simulink model "main_commande"  (R2024b)
settings: Solver=FixedStepAuto  StartTime=0.0  StopTime=10.0  MaxStep=0.01  RelTol=1e-3
undefined symbols (not defined in the file or in its folder): Cf, Cr, e_max, epsilon, Izz, lf, lr, m, q, TV
libraries: simulink x2
settings Model: PacingRate=0.100000  Creator=marti  LastModifiedBy=Filip

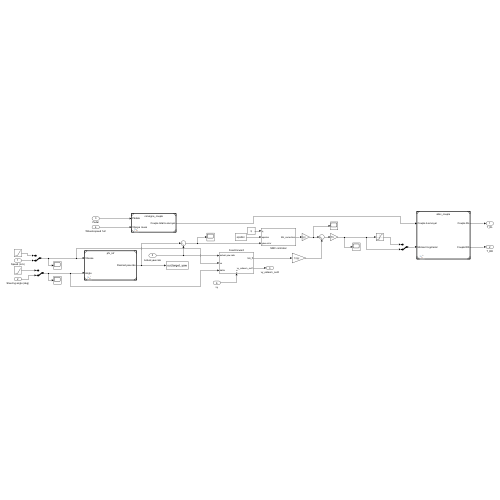
[thumbnail: Simulink's stored preview of the top-level diagram]
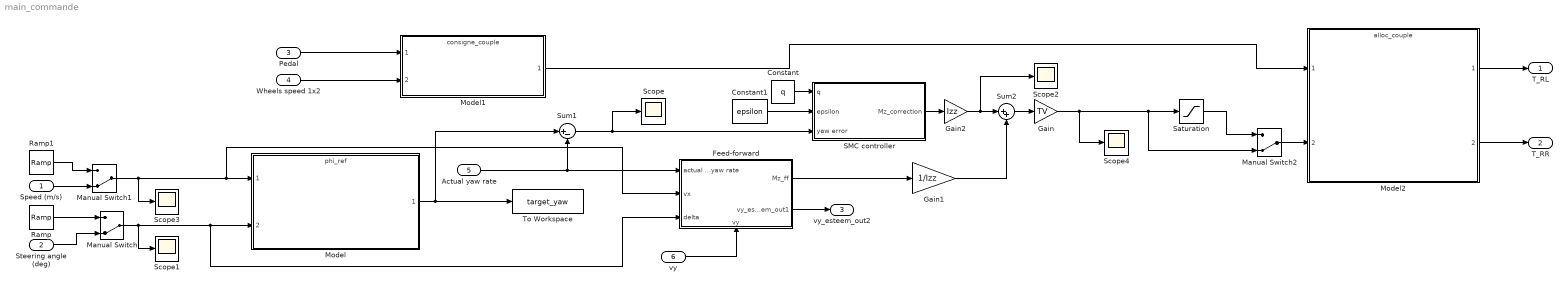
== system main_commande ==
  Speed (m/s) : Inport
  Steering angle (deg) : Inport  Port=2
  Pedal : Inport  Port=3
  Wheels speed 1x2 : Inport  Port=4
  Actual yaw rate : Inport  Port=5
  vy : Inport  Port=6
  Constant : Constant  Value=q
  Constant1 : Constant  Value=epsilon
  Feed-forward : Subsystem
      settings: PortSchema="{\"entries\":[{\"content\":{\"sides\":[{\"content\":{\"connectorIds\":[\"In1\",\"In2\",\"In3\"]},\"type\":\"ConnectorPlacement.EquallySpacedRectSide\",\"uuid\":\"af8368cf-4f84-4250-9673-79f62898b3cc\"},{\"content\":{\"connectorIds\":[\"Out1\",\"Out2\"],\"side\":\"RIGHT\"},\"type\":\"ConnectorPlacement.EquallySpacedRectSide\",\"uuid\":\"09f02962-5c7c-4455-ad81-befc240d6e55\"},{\"content\":{\"side\":\"TOP\"},\"type\":\"ConnectorPlacement.EquallySpacedRectSide\",\"uuid\":\"7a5fb401-319c-4a88-af01-2dc8b8cc2b6a\"},{\"content\":{\"connectorIds\":[\"In4\"],\"side\":\"BOTTOM\"},\"type\":\"ConnectorPlacement.EquallySpacedRectSide\",\"uuid\":\"65b1ac5c-7626-4bf0-b657-0a59cfe23dc9\"}]},\"type\":\"ConnectorPlacement.EquallySpacedConnector\",\"uuid\":\"62a1c25a-eba9-43b8-a069-759f180a4ce0\"}],\"packageUris\":[\"http://schema.mathworks.com/mf0/Connector/R2020b\"],\"version\":\"1.0\"}"
  Gain : Gain  Gain=TV
  Gain1 : Gain  Gain=1/Izz
  Gain2 : Gain  Gain=Izz
  Manual Switch : ManualSwitch  CurrentSetting=0
  Manual Switch1 : ManualSwitch  CurrentSetting=0
  Manual Switch2 : ManualSwitch  CurrentSetting=0
  Model : ModelReference  ModelNameDialog=phi_ref.slx  SimulationMode=Normal  ModelReferenceVersion=1.22
  Model1 : ModelReference  ModelNameDialog=consigne_couple.slx  SimulationMode=Normal  ModelReferenceVersion=1.13
  Model2 : ModelReference  ModelNameDialog=alloc_couple.slx  SimulationMode=Normal  ModelReferenceVersion=1.5
  Ramp : simulink/Sources/Ramp  slope=5  start=2  InitialOutput=0
  Ramp1 : simulink/Sources/Ramp  slope=10  start=0  InitialOutput=1
  SMC controller : Subsystem
  Saturation : Saturate  UpperLimit=400  LowerLimit=-400
  Scope{,1..4} (5 alike) : Scope
  Sum1 : Sum  Inputs=|+-
  Sum2 : Sum  Inputs=|++
  To Workspace : ToWorkspace  VariableName=target_yaw  SaveFormat=Structure With Time  SampleTime=-1
  T_RL : Outport
  T_RR : Outport  Port=2
  vy_esteem_out2 : Outport  Port=3
  wires:
  Gain/1 -> Scope4/1, Manual Switch2/2, Saturation/1
  Pedal/1 -> Model1/1
  Wheels speed 1x2/1 -> Model1/2
  Model2/1 -> T_RL/1
  Model2/2 -> T_RR/1
  Ramp/1 -> Manual Switch/1
  Steering angle (deg)/1 -> Manual Switch/2
  Speed (m/s)/1 -> Manual Switch1/2
  Ramp1/1 -> Manual Switch1/1
  Model/1 -> Sum1/1, To Workspace/1
  Saturation/1 -> Manual Switch2/1
  Manual Switch2/1 -> Model2/2
  Sum1/1 -> Scope/1, SMC controller/3(yaw error)
  Feed-forward/2(vy_esteem_out1) -> vy_esteem_out2/1
  Feed-forward/1(Mz_ff) -> Gain1/1
  SMC controller/1(Mz_correction) -> Gain2/1
  Gain2/1 -> Scope2/1, Sum2/1
  Constant1/1 -> SMC controller/2(epsilon)
  Constant/1 -> SMC controller/1(q)
  Actual yaw rate/1 -> Feed-forward/1(actual yaw rate), Sum1/2
  Manual Switch1/1 -> Feed-forward/2(vx), Model/1, Scope3/1
  Sum2/1 -> Gain/1
  Manual Switch/1 -> Feed-forward/3(delta), Model/2, Scope1/1
  vy/1 -> Feed-forward/4(vy)
  Model1/1 -> Model2/1
  Gain1/1 -> Sum2/2

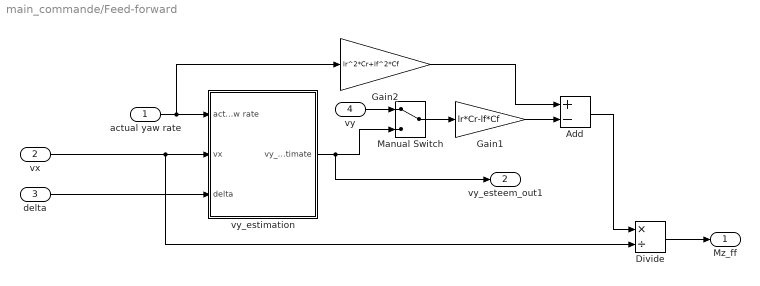
== system main_commande/Feed-forward ==
  actual yaw rate : Inport
  vx : Inport  Port=2
  delta : Inport  Port=3
  vy : Inport  Port=4
  Add : Sum  Inputs=+-
  Divide : Product  Inputs=*/
  Gain1 : Gain  Gain=lr*Cr-lf*Cf
  Gain2 : Gain  Gain=lr^2*Cr+lf^2*Cf
  Manual Switch : ManualSwitch
  vy_estimation : Subsystem
  Mz_ff : Outport
  vy_esteem_out1 : Outport  Port=2
  wires:
  vx/1 -> Divide/2, vy_estimation/2(vx)
  Gain2/1 -> Add/1
  delta/1 -> vy_estimation/3(delta)
  Add/1 -> Divide/1
  vy_estimation/1(vy_estimate) -> Manual Switch/2, vy_esteem_out1/1
  Divide/1 -> Mz_ff/1
  actual yaw rate/1 -> Gain2/1, vy_estimation/1(actual yaw rate)
  Gain1/1 -> Add/2
  vy/1 -> Manual Switch/1
  Manual Switch/1 -> Gain1/1

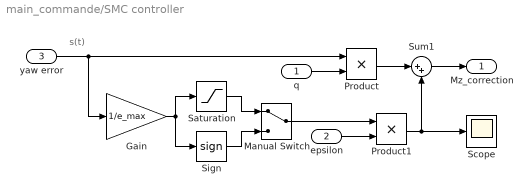
== system main_commande/SMC controller ==
  note: s(t)
  q : Inport
  epsilon : Inport  Port=2
  yaw error : Inport  Port=3
  Gain : Gain  Gain=1/e_max
  Manual Switch : ManualSwitch
  Product : Product
  Product1 : Product
  Saturation : Saturate  UpperLimit=1  LowerLimit=-1
  Scope : Scope
  Sign : Signum
  Sum1 : Sum  Inputs=|++
  Mz_correction : Outport
  wires:
  Product/1 -> Sum1/1
  Sum1/1 -> Mz_correction/1
  yaw error/1 -> Product/1, Gain/1
  q/1 -> Product/2
  epsilon/1 -> Product1/2
  Manual Switch/1 -> Product1/1
  Gain/1 -> Sign/1, Saturation/1
  Product1/1 -> Sum1/2, Scope/1
  Saturation/1 -> Manual Switch/1
  Sign/1 -> Manual Switch/2

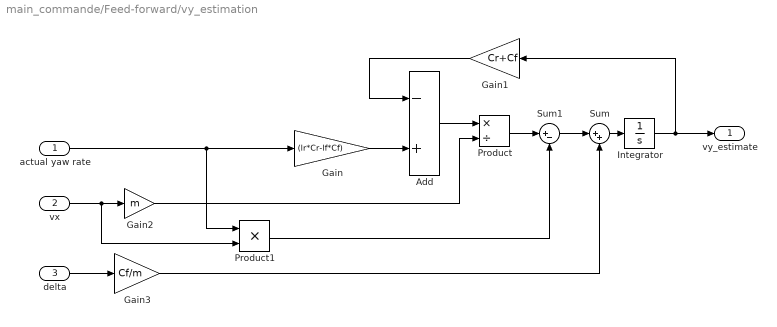
== system main_commande/Feed-forward/vy_estimation ==
  actual yaw rate : Inport
  vx : Inport  Port=2
  delta : Inport  Port=3
  Add : Sum  Inputs=-+
  Gain : Gain  Gain=(lr*Cr-lf*Cf)
  Gain1 : Gain  Gain=Cr+Cf
  Gain2 : Gain  Gain=m
  Gain3 : Gain  Gain=Cf/m
  Integrator : Integrator
  Product : Product  Inputs=*/
  Product1 : Product
  Sum : Sum  Inputs=|++
  Sum1 : Sum  Inputs=|+-
  vy_estimate : Outport
  wires:
  Integrator/1 -> vy_estimate/1, Gain1/1
  Gain/1 -> Add/2
  delta/1 -> Gain3/1
  Gain1/1 -> Add/1
  Add/1 -> Product/1
  Gain2/1 -> Product/2
  Product/1 -> Sum1/1
  vx/1 -> Product1/2, Gain2/1
  actual yaw rate/1 -> Product1/1, Gain/1
  Sum/1 -> Integrator/1
  Gain3/1 -> Sum/2
  Sum1/1 -> Sum/1
  Product1/1 -> Sum1/2
